simulink model "FSModem"  (R2017b)
settings: Solver=FixedStepDiscrete  StartTime=0.0  StopTime=10.0  RelTol=1e-3
InitFcn:
  | theta = 0:pi/4:(2*pi)-(pi/4);
  | Fs_8 = cos(theta) +i*sin(theta);
  | sample_time = 1/1e6;
undefined symbols (not defined in the file): i
libraries: hdlsllib x2
settings Model: DataTypeOverride=Off  Creator=ppradhan  LastModifiedBy=ppradhan
settings DataIOCC: SaveOutput=off  SaveTime=off
settings OptimizationCC: BlockReduction=off  ConditionallyExecuteInputs=off  DefaultParameterBehavior=Inlined
settings DebuggingCC: AlgebraicLoopMsg=error  SingleTaskRateTransMsg=error  StrictBusMsg=ErrorOnBusTreatedAsVector
settings HardwareCC: ProdBitPerPointer=32  ProdBitPerSizeT=32  ProdBitPerPtrDiffT=32  ProdLargestAtomicFloat=None  ProdIntDivRoundTo=Undefined  ProdEndianess=Unspecified  ProdWordSize=32  ProdHWDeviceType=ASIC/FPGA->ASIC/FPGA  ProdEqTarget=off
settings CodeAppCC: StateflowObjectComments=on

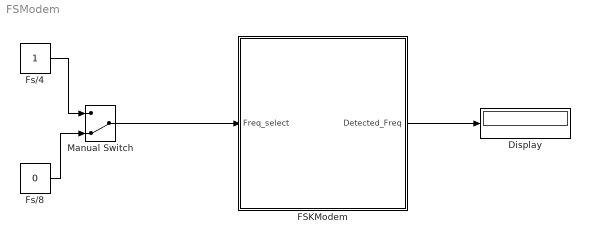
== system FSModem ==
  Display : Display
  FSKModem : Subsystem
  Fs/4 : Constant  OutDataTypeStr=boolean  SampleTime=sample_time
  Fs/8 : Constant  Value=0  OutDataTypeStr=boolean  SampleTime=sample_time
  Manual Switch : ManualSwitch  CurrentSetting=0
  wires:
  FSKModem/1(Detected_Freq) -> Display/1
  Manual Switch/1 -> FSKModem/1(Freq_select)
  Fs/4/1 -> Manual Switch/1
  Fs/8/1 -> Manual Switch/2

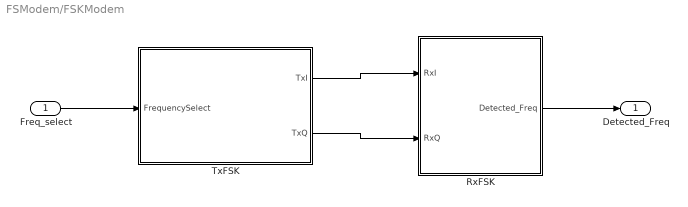
== system FSModem/FSKModem ==
  Freq_select : Inport
  RxFSK : Subsystem
  TxFSK : Subsystem
  Detected_Freq : Outport
  wires:
  Freq_select/1 -> TxFSK/1(FrequencySelect)
  RxFSK/1(Detected_Freq) -> Detected_Freq/1
  TxFSK/2(TxQ) -> RxFSK/2(RxQ)
  TxFSK/1(TxI) -> RxFSK/1(RxI)

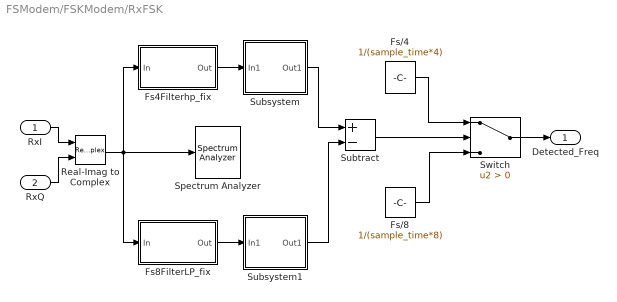
== system FSModem/FSKModem/RxFSK ==
  RxI : Inport
  RxQ : Inport  Port=2
  Fs/4 : Constant  Value=1/(sample_time*4)  OutDataTypeStr=fixdt(1,16)  SampleTime=sample_time
  Fs/8 : Constant  Value=1/(sample_time*8)  OutDataTypeStr=fixdt(1,16)  SampleTime=sample_time
  Fs4Filterhp_fix : Subsystem  Tag=BlockMethodSubSystem
  Fs8FilterLP_fix : Subsystem  Tag=BlockMethodSubSystem
  Real-Imag to Complex : RealImagToComplex
  Spectrum Analyzer : SpectrumAnalyzer
  Subsystem : Subsystem
  Subsystem1 : Subsystem
  Subtract : Sum  Inputs=+-
  Switch : Switch  Criteria=u2 > Threshold
  Detected_Freq : Outport
  wires:
  Subsystem/1(Out1) -> Subtract/1
  Subtract/1 -> Switch/2
  Fs/4/1 -> Switch/1
  Fs/8/1 -> Switch/3
  Switch/1 -> Detected_Freq/1
  Subsystem1/1(Out1) -> Subtract/2
  Fs8FilterLP_fix/1(Out) -> Subsystem1/1(In1)
  Fs4Filterhp_fix/1(Out) -> Subsystem/1(In1)
  RxI/1 -> Real-Imag to Complex/1
  RxQ/1 -> Real-Imag to Complex/2
  Real-Imag to Complex/1 -> Fs8FilterLP_fix/1(In), Fs4Filterhp_fix/1(In), Spectrum Analyzer/1

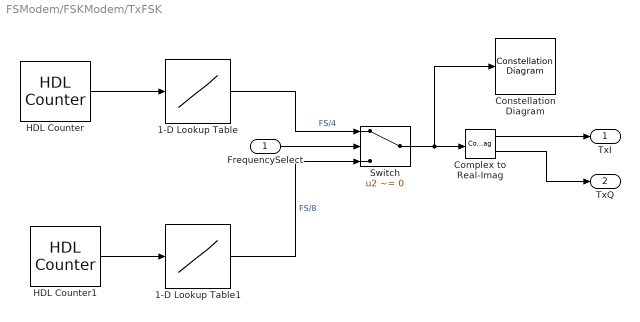
== system FSModem/FSKModem/TxFSK ==
  FrequencySelect : Inport
  1-D Lookup Table : Lookup_n-D  NumberOfTableDimensions=1  BreakpointsForDimension1=[0:3]  BreakpointsForDimension1FirstPoint=10  BreakpointsForDimension2FirstPoint=10  BreakpointsForDimension1Spacing=12  BreakpointsForDimension2Spacing=12  IndexSearchMethod=Evenly spaced points  Table=[1+0*i, 0+i,-1+0*i, 0-i]  TableDataTypeStr=fixdt(1,16,14)  InterpMethod=Flat  DiagnosticForOutOfRangeInput=Error  InternalRulePriority=Speed  OutDataTypeStr=fixdt(1,16,14)  RndMeth=Simplest  InputSameDT=on
  1-D Lookup Table1 : Lookup_n-D  NumberOfTableDimensions=1  BreakpointsForDimension1=[0:7]  BreakpointsForDimension1FirstPoint=10  BreakpointsForDimension2FirstPoint=10  BreakpointsForDimension1Spacing=12  BreakpointsForDimension2Spacing=12  IndexSearchMethod=Evenly spaced points  Table=Fs_8  TableDataTypeStr=fixdt(1,16,14)  InterpMethod=Flat  DiagnosticForOutOfRangeInput=Error  InternalRulePriority=Speed  OutDataTypeStr=fixdt(1,16,14)  RndMeth=Simplest  InputSameDT=on
  Complex to Real-Imag : ComplexToRealImag
  Constellation Diagram : ConstellationDiagram
  HDL Counter : hdlsllib/HDL Operations/HDL Counter  CountType=Free running  CountInit=0  CountStep=1  CountMax=25  CountFromType=Initial value  CountFrom=0  CountResetPort=off  CountLoadPort=off  CountEnbPort=off  CountDirPort=off  CountDataType=Unsigned  CountWordLen=2  CountFracLen=0  CountSampTime=sample_time
      settings: SourceProductName=HDL Coder  SourceProductBaseCode=HD
  HDL Counter1 : hdlsllib/HDL Operations/HDL Counter  CountType=Free running  CountInit=0  CountStep=1  CountMax=25  CountFromType=Initial value  CountFrom=0  CountResetPort=off  CountLoadPort=off  CountEnbPort=off  CountDirPort=off  CountDataType=Unsigned  CountWordLen=3  CountFracLen=0  CountSampTime=sample_time
      settings: SourceProductName=HDL Coder  SourceProductBaseCode=HD
  Switch : Switch  Criteria=u2 ~= 0
  TxI : Outport
  TxQ : Outport  Port=2
  wires:
  1-D Lookup Table/1 -> Switch/1  "FS/4"
  HDL Counter1/1 -> 1-D Lookup Table1/1
  FrequencySelect/1 -> Switch/2
  1-D Lookup Table1/1 -> Switch/3  "FS/8"
  HDL Counter/1 -> 1-D Lookup Table/1
  Switch/1 -> Constellation Diagram/1, Complex to Real-Imag/1
  Complex to Real-Imag/1 -> TxI/1
  Complex to Real-Imag/2 -> TxQ/1

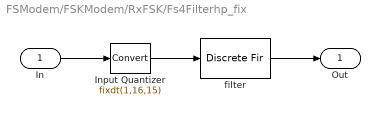
== system FSModem/FSKModem/RxFSK/Fs4Filterhp_fix ==
  In : Inport
  Input Quantizer : DataTypeConversion  OutDataTypeStr=fixdt(1,16,15)  RndMeth=Round  SaturateOnIntegerOverflow=on
  filter : DiscreteFir  Coefficients=[0.0013343852178826865 -0.037208942498876921 0.0096591102849806244 0.060294949982258796 0.044994895945192195 -0.096576041962710787 -0.2938256195866174 0.61241243421292701 -0.2938256195866174 -0.096576041962710787 0.044994895945192195 0.060294949982258796 0.0096591102849806244 -0.037208942498876921 0.0013343852178826865]  InputProcessing=Columns as channels (frame based)  CoefDataTypeStr=fixdt(true,16,15)  ProductDataTypeStr=fixdt(true,31,30)  AccumDataTypeStr=fixdt(true,32,30)  OutDataTypeStr=fixdt(true,16,15)  RndMeth=Convergent
  Out : Outport
  wires:
  In/1 -> Input Quantizer/1
  Input Quantizer/1 -> filter/1
  filter/1 -> Out/1

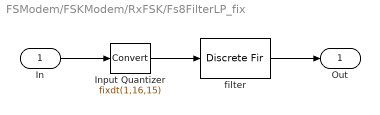
== system FSModem/FSKModem/RxFSK/Fs8FilterLP_fix ==
  In : Inport
  Input Quantizer : DataTypeConversion  OutDataTypeStr=fixdt(1,16,15)  RndMeth=Round  SaturateOnIntegerOverflow=on
  filter : DiscreteFir  Coefficients=[-0.0036634264370219907 -0.041218015500331405 -0.060716264187842602 -0.014844055350270549 0.12014351880942774 0.27886982134886168 0.35020150103238695 0.27886982134886168 0.12014351880942774 -0.014844055350270549 -0.060716264187842602 -0.041218015500331405 -0.0036634264370219907]  InputProcessing=Columns as channels (frame based)  CoefDataTypeStr=fixdt(true,16,16)  ProductDataTypeStr=fixdt(true,31,31)  AccumDataTypeStr=fixdt(true,33,31)  OutDataTypeStr=fixdt(true,16,15)  RndMeth=Convergent
  Out : Outport
  wires:
  In/1 -> Input Quantizer/1
  Input Quantizer/1 -> filter/1
  filter/1 -> Out/1

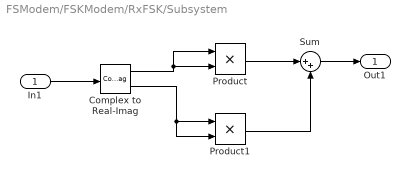
== system FSModem/FSKModem/RxFSK/Subsystem ==
  In1 : Inport
  Complex to Real-Imag : ComplexToRealImag
  Product : Product
  Product1 : Product
  Sum : Sum  Inputs=|++
  Out1 : Outport
  wires:
  In1/1 -> Complex to Real-Imag/1
  Complex to Real-Imag/1 -> Product/2, Product/1
  Product/1 -> Sum/1
  Complex to Real-Imag/2 -> Product1/2, Product1/1
  Product1/1 -> Sum/2
  Sum/1 -> Out1/1

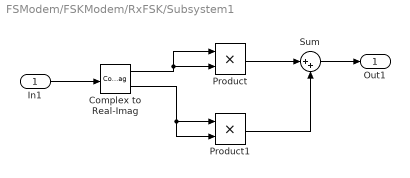
== system FSModem/FSKModem/RxFSK/Subsystem1 ==
  In1 : Inport
  Complex to Real-Imag : ComplexToRealImag
  Product : Product
  Product1 : Product
  Sum : Sum  Inputs=|++
  Out1 : Outport
  wires:
  Sum/1 -> Out1/1
  Product1/1 -> Sum/2
  Complex to Real-Imag/2 -> Product1/1, Product1/2
  Product/1 -> Sum/1
  Complex to Real-Imag/1 -> Product/1, Product/2
  In1/1 -> Complex to Real-Imag/1
